simulink model "configurationExample"  (R2019a)
settings: Solver=VariableStepAuto  StartTime=0.0  StopTime=10.0  RelTol=1e-3
settings Model: OrderedModelArguments=off  Creator=jnicholson  LastModifiedBy=jnicholson

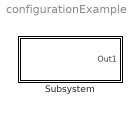
== system configurationExample ==
  Subsystem : Subsystem  mask{optionA=5, optionB=3, isOptionCenabled=off, optionC=0, optionD=59, optionE=22, optionF=20}
      mask prompts: optionA "Option A"; optionB "Option B"; isOptionCenabled "Enable Option C"; optionC "Option C"; optionD "Option D"; optionE "Option E"; optionF "Option F"
      mask TypeOptions optionA: 1 | 2 | 3 | 4 | 5
      mask Callback optionA: optionA(gcbh)
      mask TypeOptions optionB: 1 | 2 | 3 | 4
      mask Callback isOptionCenabled: isOptionCenabled(gcbh)
      mask TypeOptions optionD: 3 | 5 | 6 | 7 | 11 | 29 | 30 | 31 | 46 | 56 | 57 | 59 | 60 | 61 | 62 | 63 | 64
      mask Callback optionD: optionD(gcbh)
      mask TypeOptions optionE: 1 | 2 | 3 | 4 | 5 | 6 | 7 | 8 | 9 | 10 | 11 | 12 | 13 | 14 | 15 | 16 | 17 | 18 | 19 | 20 | 21 | 22
      mask TypeOptions optionF: 1 | 2 | 3 | 4 | 5 | 6 | 7 | 8 | 9 | 10 | 11 | 12 | 13 | 14 | 15 | 16 | 17 | 18 | 19 | 20 | 21 | 22 | 23 | 24 | 25 | 26 | 27 | 28 | 29 | 30 | 31

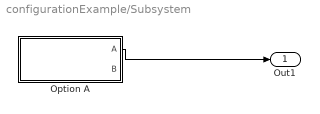
== system configurationExample/Subsystem ==
  Option A : Subsystem  VariantControlMode=Label  Variant=on  LabelModeActiveChoice=ModelA1
  Out1 : Outport
  wires:
  Option A/1(A) -> Out1/1

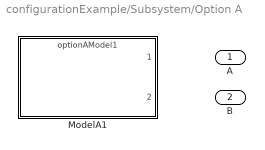
== system configurationExample/Subsystem/Option A ==
  ModelA1 : ModelReference  ModelNameDialog=optionAModel1.slx  ParameterArgumentNames=optionB  ParameterArgumentValues=optionB  UsingDefaultArgumentValue=0  SimulationMode=Normal  VariantControl=ModelA1  ModelReferenceVersion=1.11  optionB=str2double(optionB)  SimulationMode=Normal
  A : Outport
  B : Outport  Port=2
